simulink model "WPT_system_experimental_setup"  (R2022b)
settings: Solver=VariableStepAuto  StartTime=0.0  StopTime=0.030  RelTol=1e-3  EnableMultiTasking=on
InitFcn:
  | % Global param
  | f0 = 85000;
  | V_dc = 10;
  | Max_c = 5;
  | rise_time = 3e-3;
  | 
  | % Zed board ADC param
  | ADC_max_amp = 40;
  | ADC_max_vol = 1.25;
  | ADC_f_sample = 1e6;
  | ADC_bits = 12;
  | 
  | % Primary param
  | L1 = 24e-6;
  | C1 = 138e-9; %1/((2*pi*f0)^2*L1);
  | R1 = 0.075;
  | 
  | 
  | % Secondary param
  | M = 1.6e-6;
  | L2 = 24e-6;
  | C2 = 141e-9;% 1/((2*pi*f0)^2*L2);
  | 
  | R2 = 0.075;
  | R_l = 1.25;
  | C_out = 10e-6;
  | L_out = 1e-6;
  | 
  | % PRBS param
  | PRBS_n_bit = 10;
  | PRBS_f = f0*2; %1e5;
  | PRBS_up = 1; % pwm up time in %
  | PRBS_delay = 1.1* 1/(PRBS_f) * PRBS_up/100;
  | PRBS_amplitude = 0.1;
  | PRBS_n_period = 2;
  | PRBS_t_start = 0.0002 + PRBS_n_period * (2^(PRBS_n_bit) - 1)/PRBS_f;
  | PRBS_t_stop = 0.0002 + 2*PRBS_n_period * (2^(PRBS_n_bit) - 1)/PRBS_f;
  | transport_delay = PRBS_t_stop - PRBS_t_start;
  | 
  | 
  | % Emphasis filters param
  | 
  | f_z = 42000;
  | T_s_1 = 1/PRBS_f;
  | T_s_2 = 1/ADC_f_sample;
  | Filter_param_1 = exp(-2*pi*T_s_1 * f_z);
  | Filter_param_2 = exp(-2*pi*T_s_2 * f_z);
  | 
  | %Filter_param = 0.652296150979446; % 68000
model workspace (MAT data in the model file):
  C1 = Simulink.Parameter
  C1.Value = 4.1e-08
  C1.DataType = 'auto'
  C1.Complexity = 'real'
  C1.Dimensions = [1 1]
  C2 = Simulink.Parameter
  C2.Value = 4.2e-08
  C2.DataType = 'auto'
  C2.Complexity = 'real'
  C2.Dimensions = [1 1]
  C_out = Simulink.Parameter
  C_out.Value = 1e-05
  C_out.DataType = 'auto'
  C_out.Complexity = 'real'
  C_out.Dimensions = [1 1]
  L1 = Simulink.Parameter
  L1.Value = 8.6e-05
  L1.DataType = 'auto'
  L1.Complexity = 'real'
  L1.Dimensions = [1 1]
  L2 = Simulink.Parameter
  L2.Value = 8.4e-05
  L2.DataType = 'auto'
  L2.Complexity = 'real'
  L2.Dimensions = [1 1]
  M = Simulink.Parameter
  M.Value = 7e-06
  M.DataType = 'auto'
  M.Complexity = 'real'
  M.Dimensions = [1 1]
  R1 = Simulink.Parameter
  R1.Value = 0.35
  R1.DataType = 'auto'
  R1.Complexity = 'real'
  R1.Dimensions = [1 1]
  R2 = Simulink.Parameter
  R2.Value = 0.3
  R2.DataType = 'auto'
  R2.Complexity = 'real'
  R2.Dimensions = [1 1]
  R_l = Simulink.Parameter
  R_l.Value = 2
  R_l.DataType = 'auto'
  R_l.Complexity = 'real'
  R_l.Dimensions = [1 1]
  V_dc = Simulink.Parameter
  V_dc.Value = 400
  V_dc.DataType = 'auto'
  V_dc.Complexity = 'real'
  V_dc.Dimensions = [1 1]
  f0 = Simulink.Parameter
  f0.Value = 85000
  f0.DataType = 'auto'
  f0.Complexity = 'real'
  f0.Dimensions = [1 1]
  mwTaskManagerKernelLatency = 0
undefined symbols (not defined in the file or in its folder): plecs
libraries: simulink_extras x36, simulink x6, hdlsllib x3, msbAdcArchitectures x2, plecslib_extras2 x2, slpidlib x2
CloseFcn:
  | % Define the command to call the Python script
  | pythonScript = 'cross_correlation.py';
  | command = ['python ', pythonScript];
  | 
  | % Execute the Python script
  | system(command);
settings Model: Creator=thoma  LastModifiedBy=thoma
settings SolverCC: PositivePriorityOrder=on
settings OptimizationCC: EnhancedBackFolding=on  PassReuseOutputArgsAs=Individual arguments  ZeroExternalMemoryAtStartup=off  ZeroInternalMemoryAtStartup=off  MaxStackSize=64  OptimizeBlockOrder=speed  DifferentSizesBufferReuse=on  OptimizationCustomize=off  EfficientTunableParamExpr=on
settings DebuggingCC: ParameterTunabilityLossMsg=error
settings HardwareCC: ProdBitPerPointer=32  ProdBitPerSizeT=32  ProdBitPerPtrDiffT=32  ProdLargestAtomicInteger=Long  ProdLargestAtomicFloat=Double  ProdWordSize=32  ProdHWDeviceType=ARM Compatible->ARM Cortex  HardwareBoardFeatureSet=SoCBlockset
settings ModelReferenceCC: ModelReferenceNumInstancesAllowed=Single
settings SFSimCC: MATLABDynamicMemAlloc=off
settings RTWCC: Description=Embedded Coder  SystemTargetFile=ert.tlc  HardwareBoard=ZedBoard  TLCOptions="-aInlineSetEventsForThisBaseRateFcn=TLC_FALSE -aSuppressMultiTaskScheduler=TLC_FALSE  -aRateBasedStepFcn=0"  TemplateMakefile=ert_default_tmf
settings CodeAppCC: ForceParamTrailComments=on  IgnoreCustomStorageClasses=off  OperatorAnnotations=on  SimulinkDataObjDesc=on  SFDataObjDesc=on  InsertBlockDesc=on

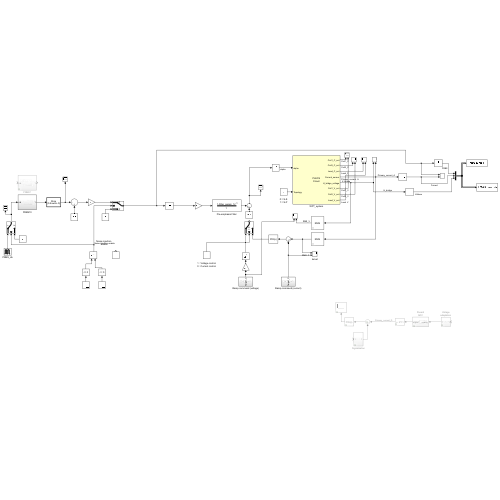
[thumbnail: Simulink's stored preview of the top-level diagram]
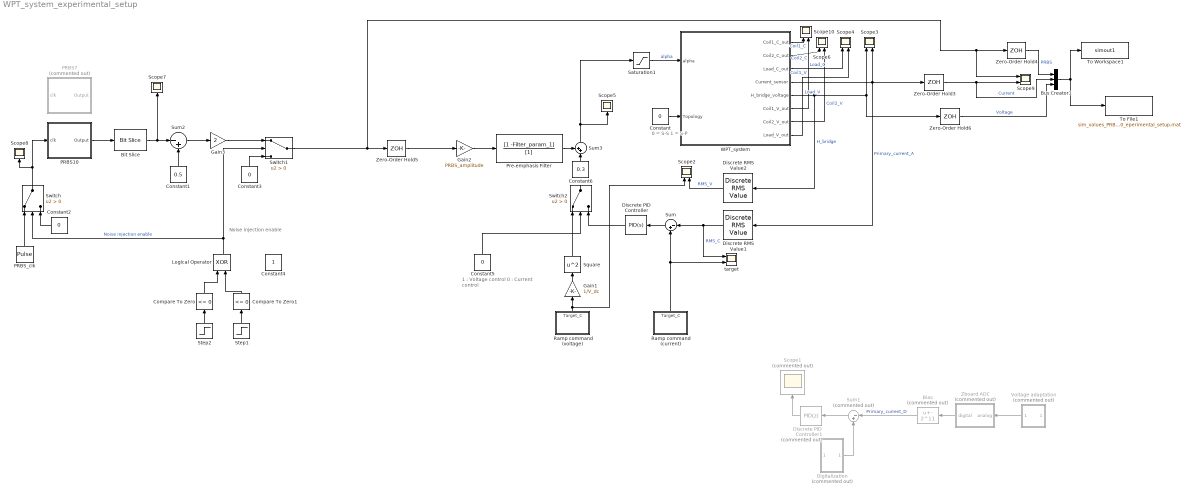
== system WPT_system_experimental_setup ==
  note: 0 = S-S
      | 1 = S-P
  note: Noise injection
      | enable
  note: 1 : Voltage control
      | 0 : Current control
  Bias : Bias  Commented=on  Bias=- 2^11  SaturateOnIntegerOverflow=off
  Bit Slice : hdlsllib/Logic and Bit Operations/Bit Slice  lidx=0  ridx=0
  Bus Creator1 : BusCreator  Inputs=3
  Compare To Zero : simulink/Logic and Bit Operations/Compare To Zero  relop=<=  OutDataTypeStr=boolean
  Compare To Zero1 : simulink/Logic and Bit Operations/Compare To Zero  relop=<=  OutDataTypeStr=boolean
  Constant{,2..3,5} (4 alike) : Constant  Value=0
  Constant1 : Constant  Value=0.5
  Constant4 : Constant
  Constant6 : Constant  Value=0.3
  Digitalization : Subsystem  Commented=on
  Discrete RMS Value1 : plecslib_extras2/Discrete Analysis/Discrete RMS Value  init=0  Ts=1/(30 * f0)  samples=60
      settings: SourceProductName=PLECS Extras
  Discrete RMS Value2 : plecslib_extras2/Discrete Analysis/Discrete RMS Value  init=0  Ts=1/(400 * f0)  samples=400
      settings: SourceProductName=PLECS Extras
  Discrete PID Controller : slpidlib/PID Controller  Controller=PID  Form=Parallel  TimeDomain=Continuous-time  UseExternalTs=off  SampleTime=-1  IntegratorMethod=Forward Euler  FilterMethod=Forward Euler  ControllerParametersSource=internal  P=0.075  I=5000  UseKiTs=off  D=0  N=100  UseFilter=on  TunerSelectOption=Transfer Function Based (PID Tuner App)  InitialConditionSource=internal  InitialConditionForIntegrator=0  InitialConditionForFilter=0  DifferentiatorICPrevScaledInput=0  ExternalReset=none  TrackingMode=off  Kt=1  LimitOutput=off  SatLimitsSource=internal  UpperSaturationLimit=inf  LowerSaturationLimit=-inf  LinearizeAsGain=off  AntiWindupMode=none  Kb=1  LimitIntegrator=off  UpperIntegratorSaturationLimit=inf  LowerIntegratorSaturationLimit=-inf  POutMin=[]  POutMax=[]  IOutMin=[]  IOutMax=[]  DOutMin=[]  DOutMax=[]  NOutMin=[]  NOutMax=[]  SumOutMin=[]  SumOutMax=[]  SaturationOutMin=[]  SaturationOutMax=[]  PParamMin=[]  PParamMax=[]  IParamMin=[]  IParamMax=[]  DParamMin=[]  DParamMax=[]  NParamMin=[]  NParamMax=[]  KbParamMin=[]  KbParamMax=[]  KtParamMin=[]  KtParamMax=[]  KbOutMin=[]  KbOutMax=[]  KtOutMin=[]  KtOutMax=[]  IntegratorOutMin=[]  IntegratorOutMax=[]  FilterOutMin=[]  FilterOutMax=[]  SumI1OutMin=[]  SumI1OutMax=[]  SumI2OutMin=[]  SumI2OutMax=[]  SumI3OutMin=[]  SumI3OutMax=[]  SumI4OutMin=[]  SumI4OutMax=[]  SumDOutMin=[]  SumDOutMax=[]  DifferentiatorOutMin=[]  DifferentiatorOutMax=[]  FilterDiffOutCoefMin=[]  FilterDiffOutCoefMax=[]  ReciprocalOutMin=[]  ReciprocalOutMax=[]  SumDenOutMin=[]  SumDenOutMax=[]  SumNumOutMin=[]  SumNumOutMax=[]  DivideOutMin=[]  DivideOutMax=[]  UdiffTsProdOutMin=[]  UdiffTsProdOutMax=[]  NTsProdOutMin=[]  NTsProdOutMax=[]  UintegralTsProdOutMin=[]  UintegralTsProdOutMax=[]  UngainTsProdOutMin=[]  UngainTsProdOutMax=[]  ClampingZeroOutDataTypeStr=Inherit: Inherit via back propagation  ClampingZeroOutMin=[]  ClampingZeroOutMax=[]  FilterDenConstantOutDataTypeStr=Inherit: Inherit via back propagation  FilterDenConstantOutMin=[]  FilterDenConstantOutMax=[]  PCopyOutDataTypeStr=Inherit: Inherit via back propagation  PCopyOutMin=[]  PCopyOutMax=[]  NCopyOutDataTypeStr=Inherit: Inherit via back propagation  NCopyOutMin=[]  NCopyOutMax=[]  IntegratorContinuousStateAttributes=''  IntegratorStateMustResolveToSignalObject=off  IntegratorRTWStateStorageClass=Auto  FilterContinuousStateAttributes=''  FilterStateMustResolveToSignalObject=off  FilterRTWStateStorageClass=Auto  ParallelPVariant=InternalParameters  IdealPVariant=Disabled  IVariant=InternalParameters  DVariant=InternalParameters  IntegratorVariant=Continuous  SatVariant=Disabled  AWVariant=Passthrough  PCopyVariant=Disabled  TRVariant=Disabled  FdbkBlocksVariant=Forward  IdealPFdbkVariant=Disabled  SatFdbkVariant=Disabled  DerivativeFilterVariant=ContFilter  NVariant=InternalParameters  NCopyVariant=Disabled  FilterICVariant=InternalICsFilter  IntegratorICVariant=InternalICs  ExternalResetVariant=Disabled  TRSumVariant=Passthrough  SumFdbkVariant=Disabled  SumVariant=Sum_PID  TsampFilterVariant=InternalTs  TsampNgainVariant=Passthrough  TsampIntegralVariant=Passthrough  ExternalSaturationOutDataTypeStr=Inherit: Same as second input
      settings: LibrarySourceBlock=hdlsllib/Discrete/Discrete PID Controller
  Discrete PID Controller1 : slpidlib/PID Controller  Commented=on  Controller=PID  Form=Parallel  TimeDomain=Discrete-time  UseExternalTs=off  SampleTime=-1  IntegratorMethod=Forward Euler  FilterMethod=Forward Euler  ControllerParametersSource=internal  P=24  I=0  UseKiTs=off  D=0  N=100  UseFilter=on  TunerSelectOption=Transfer Function Based (PID Tuner App)  InitialConditionSource=internal  InitialConditionForIntegrator=0  InitialConditionForFilter=0  DifferentiatorICPrevScaledInput=0  ExternalReset=none  TrackingMode=off  Kt=1  LimitOutput=off  SatLimitsSource=internal  UpperSaturationLimit=inf  LowerSaturationLimit=-inf  LinearizeAsGain=off  AntiWindupMode=none  Kb=1  LimitIntegrator=off  UpperIntegratorSaturationLimit=inf  LowerIntegratorSaturationLimit=-inf  POutMin=[]  POutMax=[]  IOutMin=[]  IOutMax=[]  DOutMin=[]  DOutMax=[]  NOutMin=[]  NOutMax=[]  SumOutMin=[]  SumOutMax=[]  SaturationOutMin=[]  SaturationOutMax=[]  PParamMin=[]  PParamMax=[]  IParamMin=[]  IParamMax=[]  DParamMin=[]  DParamMax=[]  NParamMin=[]  NParamMax=[]  KbParamMin=[]  KbParamMax=[]  KtParamMin=[]  KtParamMax=[]  KbOutMin=[]  KbOutMax=[]  KtOutMin=[]  KtOutMax=[]  IntegratorOutMin=[]  IntegratorOutMax=[]  FilterOutMin=[]  FilterOutMax=[]  SumI1OutMin=[]  SumI1OutMax=[]  SumI2OutMin=[]  SumI2OutMax=[]  SumI3OutMin=[]  SumI3OutMax=[]  SumI4OutMin=[]  SumI4OutMax=[]  SumDOutMin=[]  SumDOutMax=[]  DifferentiatorOutMin=[]  DifferentiatorOutMax=[]  FilterDiffOutCoefMin=[]  FilterDiffOutCoefMax=[]  ReciprocalOutMin=[]  ReciprocalOutMax=[]  SumDenOutMin=[]  SumDenOutMax=[]  SumNumOutMin=[]  SumNumOutMax=[]  DivideOutMin=[]  DivideOutMax=[]  UdiffTsProdOutMin=[]  UdiffTsProdOutMax=[]  NTsProdOutMin=[]  NTsProdOutMax=[]  UintegralTsProdOutMin=[]  UintegralTsProdOutMax=[]  UngainTsProdOutMin=[]  UngainTsProdOutMax=[]  ClampingZeroOutDataTypeStr=Inherit: Inherit via back propagation  ClampingZeroOutMin=[]  ClampingZeroOutMax=[]  FilterDenConstantOutDataTypeStr=Inherit: Inherit via back propagation  FilterDenConstantOutMin=[]  FilterDenConstantOutMax=[]  PCopyOutDataTypeStr=Inherit: Inherit via back propagation  PCopyOutMin=[]  PCopyOutMax=[]  NCopyOutDataTypeStr=Inherit: Inherit via back propagation  NCopyOutMin=[]  NCopyOutMax=[]  IntegratorContinuousStateAttributes=''  IntegratorStateMustResolveToSignalObject=off  IntegratorRTWStateStorageClass=Auto  FilterContinuousStateAttributes=''  FilterStateMustResolveToSignalObject=off  FilterRTWStateStorageClass=Auto  ParallelPVariant=InternalParameters  IdealPVariant=Disabled  IVariant=InternalParameters  DVariant=InternalParameters  IntegratorVariant=Discrete  SatVariant=Disabled  AWVariant=Passthrough  PCopyVariant=Disabled  TRVariant=Disabled  FdbkBlocksVariant=Forward  IdealPFdbkVariant=Disabled  SatFdbkVariant=Disabled  DerivativeFilterVariant=ForwardEulerFilter  NVariant=InternalParameters  NCopyVariant=Disabled  FilterICVariant=InternalICsFilter  IntegratorICVariant=InternalICs  ExternalResetVariant=Disabled  TRSumVariant=Passthrough  SumFdbkVariant=Disabled  SumVariant=Sum_PID  TsampFilterVariant=InternalTs  TsampNgainVariant=Passthrough  TsampIntegralVariant=Passthrough  ExternalSaturationOutDataTypeStr=Inherit: Same as second input
      settings: LibrarySourceBlock=hdlsllib/Discrete/Discrete PID Controller
  Gain1 : Gain  Gain=1/V_dc
  Gain2 : Gain  Gain=PRBS_amplitude
  Gain3 : Gain  Gain=2
  Logical Operator : Logic  Operator=XOR  AllPortsSameDT=off  OutDataTypeStr=boolean
  PRBS10 : Subsystem
  PRBS7 : Subsystem  Commented=on
  "PRBS_clk " : DiscretePulseGenerator  PulseType=Time based  Period=1/PRBS_f  PulseWidth=PRBS_up
  Pre-emphasis Filter : DiscreteFilter  Numerator=[1 -Filter_param_1]  Denominator=[1]
  Ramp command (current) : Subsystem
  Ramp command (voltage) : Subsystem
  Saturation1 : Saturate  UpperLimit=1  LowerLimit=0
  Scope1 : Scope  Commented=on
  Scope{2..4,6,9..10} (6 alike) : Scope  NumInputPorts=2
  Scope5 : Scope
  Scope7 : Scope
  Scope8 : Scope
  Square : Math  Operator=square  SignedPower=on  RndMeth=Zero
  Step1 : Step  Time=PRBS_t_start  Before=1  After=0  SampleTime=0
  Step2 : Step  Time=PRBS_t_stop  Before=1  After=0  SampleTime=0
  Sum : Sum  Inputs=|-+
  Sum1 : Sum  Commented=on  Inputs=|-+
  Sum2 : Sum  Inputs=|-+  AccumDataTypeStr=double
  Sum3 : Sum  Inputs=++|
  Switch : Switch  Criteria=u2 > Threshold  SaturateOnIntegerOverflow=off  InputSameDT=off
  Switch1 : Switch  Criteria=u2 > Threshold  SaturateOnIntegerOverflow=off  InputSameDT=off
  Switch2 : Switch  Criteria=u2 > Threshold  SaturateOnIntegerOverflow=off  InputSameDT=off
  To File1 : ToFile  Filename=sim_values_PRBS10_eperimental_setup.mat  MatrixName=values  SampleTime=1e-6
  To Workspace1 : ToWorkspace  VariableName=simout1  SampleTime=1e-6
  Voltage adaptation : Subsystem  Commented=on
  WPT_system : Subsystem  LoadFcn=plecs('sl', 200);  InitFcn=plecs('sl', 214);  StartFcn=plecs('sl', 208);  StopFcn=plecs('sl', 209);  mask(PlecsCircuit){PLECSData=<binary blob, 4092 chars, not shown>}
      mask prompts: PLECSData "PLECS Data (Do not delete or modify!)"
      mask init:
      | % PLACE CUSTOM INITIALIZATIONS ABOVE
      | % DO NOT REMOVE
      | plecs('sl', 215);
      | % DO NOT REMOVE
      settings: CopyFcn=plecs('sl', 203);  DeleteFcn=plecs('sl', 205);  UndoDeleteFcn=plecs('sl', 206);  PreSaveFcn=plecs('sl', 211);  PostSaveFcn=plecs('sl', 201);  NameChangeFcn=plecs('sl', 210);  DestroyFcn=plecs('sl', 207);  PreCopyFcn=plecs('sl', 216);  OpenFcn=plecs('sl', 202);  ErrorFcn=plerrorfcn
      mask Help: eval('plecs(''help'', ''qthelp:///creatingacircuit.html'')')
      mask Display: disp('PLECS\nCircuit')
  Zboard ADC : Subsystem  Commented=on
  Zero-Order Hold3 : ZeroOrderHold  SampleTime=1/ADC_f_sample
  Zero-Order Hold4 : ZeroOrderHold  SampleTime=1e-6
  Zero-Order Hold5 : ZeroOrderHold  SampleTime=1/PRBS_f
  Zero-Order Hold6 : ZeroOrderHold  SampleTime=1/ADC_f_sample
  target : Scope  NumInputPorts=2
  wires:
  Constant/1 -> WPT_system/2(Topology)
  Sum/1 -> Discrete PID Controller/1
  Discrete RMS Value1/1 -> Sum/1, target/1  "RMS_C"
  Bit Slice/1 -> Scope7/1, Sum2/1
  Ramp command (current)/1(Target_C) -> Sum/2, target/2
  Bias/1 -> Sum1/1  "Primary_current_D"
  Voltage adaptation/1(Out1) -> Zboard ADC/1(analog)
  Zboard ADC/1(digital) -> Bias/1
  Digitalization/1(Output) -> Sum1/2
  Sum1/1 -> Discrete PID Controller1/1
  Discrete PID Controller1/1 -> Scope1/1
  Ramp command (voltage)/1(Target_C) -> Scope2/1, Gain1/1
  Gain1/1 -> Square/1
  Constant1/1 -> Sum2/2
  Sum2/1 -> Gain3/1
  Saturation1/1 -> WPT_system/1(alpha)  "alpha"
  WPT_system/3(Load_C_out) -> Scope4/1  "Load_C"
  WPT_system/8(Load_V_out) -> Scope4/2  "Load_V"
  WPT_system/2(Coil2_C_out) -> Scope6/1  "Coil2_C"
  WPT_system/7(Coil2_V_out) -> Scope6/2  "Coil2_V"
  Square/1 -> Switch2/1
  Discrete PID Controller/1 -> Switch2/3
  Constant5/1 -> Switch2/2
  Logical Operator/1 -> Switch/2, Switch1/2  "Noise injection enable"
  "PRBS_clk "/1 -> Switch/1
  Constant2/1 -> Switch/3
  Constant3/1 -> Switch1/3
  Gain3/1 -> Switch1/1
  Discrete RMS Value2/1 -> Scope2/2  "RMS_V"
  Sum3/1 -> Scope5/1, Saturation1/1
  PRBS10/1(Output) -> Bit Slice/1
  Switch/1 -> PRBS10/1(clk), Scope8/1
  Constant6/1 -> Sum3/2
  Step2/1 -> Compare To Zero/1
  Step1/1 -> Compare To Zero1/1
  Compare To Zero/1 -> Logical Operator/1
  Compare To Zero1/1 -> Logical Operator/2
  Pre-emphasis Filter/1 -> Sum3/1
  Gain2/1 -> Pre-emphasis Filter/1
  Zero-Order Hold5/1 -> Gain2/1
  Bus Creator1/1 -> To File1/1, To Workspace1/1
  Zero-Order Hold6/1 -> Bus Creator1/3  "Voltage"
  WPT_system/5(H_bridge_voltage) -> Zero-Order Hold6/1, Scope3/1, Discrete RMS Value2/1  "H_bridge"
  Zero-Order Hold4/1 -> Bus Creator1/1  "PRBS"
  Switch1/1 -> Scope9/1, Zero-Order Hold4/1, Zero-Order Hold5/1
  Zero-Order Hold3/1 -> Bus Creator1/2, Scope9/2  "Current"
  WPT_system/4(Current_sensor) -> Zero-Order Hold3/1, Discrete RMS Value1/1, Scope3/2  "Primary_current_A"
  WPT_system/1(Coil1_C_out) -> Scope10/1  "Coil1_C"
  WPT_system/6(Coil1_V_out) -> Scope10/2  "Coil1_V"

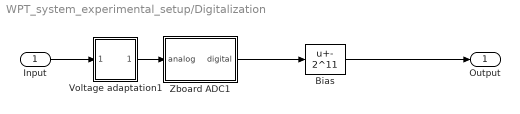
== system WPT_system_experimental_setup/Digitalization ==
  Input : Inport
  Bias : Bias  Bias=- 2^11  SaturateOnIntegerOverflow=off
  Voltage adaptation1 : Subsystem
  Zboard ADC1 : Subsystem
  Output : Outport
  wires:
  Voltage adaptation1/1(Out1) -> Zboard ADC1/1(analog)
  Input/1 -> Voltage adaptation1/1(In1)
  Zboard ADC1/1(digital) -> Bias/1
  Bias/1 -> Output/1

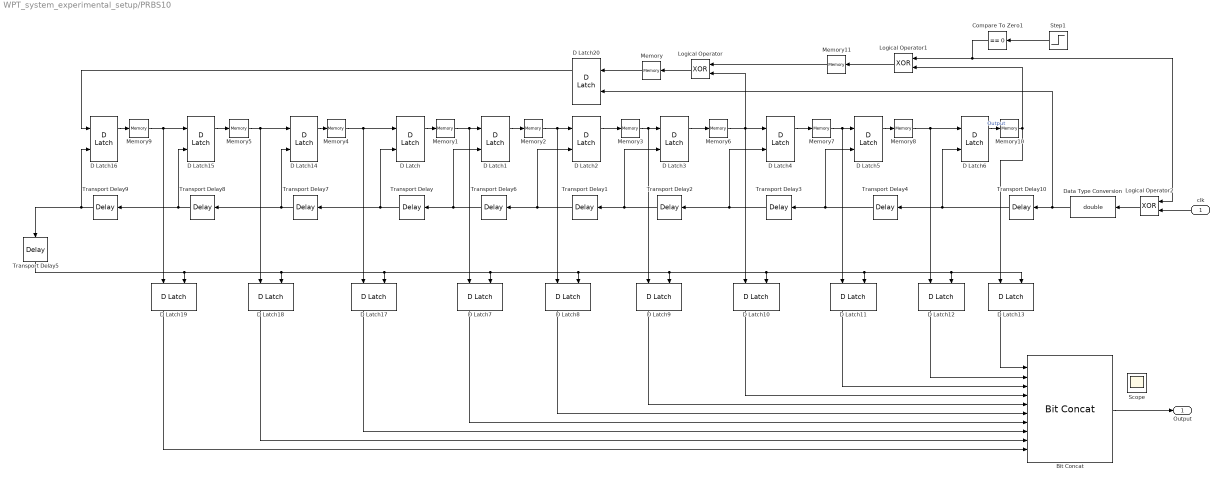
== system WPT_system_experimental_setup/PRBS10 ==
  clk : Inport
  Bit Concat : hdlsllib/Logic and Bit Operations/Bit Concat  numInputs=10
  Compare To Zero1 : simulink/Logic and Bit Operations/Compare To Zero  relop===  OutDataTypeStr=boolean
  D Latch{,1..20} (21 alike) : simulink_extras/Flip Flops/D Latch
  Data Type Conversion : DataTypeConversion  OutDataTypeStr=double  SaturateOnIntegerOverflow=off  RndMeth=Floor
  Logical Operator : Logic  Operator=XOR  AllPortsSameDT=off  OutDataTypeStr=boolean
  Logical Operator1 : Logic  Operator=XOR  AllPortsSameDT=off  OutDataTypeStr=boolean
  Logical Operator2 : Logic  Operator=XOR  AllPortsSameDT=off
  Memory{,1..11} (12 alike) : Memory
  Scope : Scope
  Step1 : Step  Time=1* PRBS_delay  SampleTime=0
  Transport Delay{,1..4,6..10} (10 alike) : TransportDelay  DelayTime=PRBS_delay  BufferSize=16384
  Transport Delay5 : TransportDelay  DelayTime=PRBS_delay  InitialOutput=1  BufferSize=16384
  Output : Outport
  wires:
  Transport Delay1/1 -> D Latch2/2, Transport Delay6/1
  Transport Delay4/1 -> D Latch5/2, Transport Delay3/1
  Transport Delay2/1 -> D Latch3/2, Transport Delay1/1
  Transport Delay3/1 -> D Latch4/2, Transport Delay2/1
  D Latch1/1 -> Memory2/1
  D Latch/1 -> Memory1/1
  D Latch2/1 -> Memory3/1
  Logical Operator/1 -> Memory/1
  D Latch4/1 -> Memory7/1
  D Latch3/1 -> Memory6/1
  Bit Concat/1 -> Output/1
  D Latch5/1 -> Memory8/1
  Transport Delay6/1 -> D Latch1/2, Transport Delay/1
  Memory3/1 -> D Latch3/1, D Latch9/1
  D Latch6/1 -> Memory10/1  "Output"
  D Latch13/1 -> Bit Concat/1
  D Latch12/1 -> Bit Concat/2
  D Latch11/1 -> Bit Concat/3
  D Latch10/1 -> Bit Concat/4
  D Latch9/1 -> Bit Concat/5
  D Latch8/1 -> Bit Concat/6
  D Latch7/1 -> Bit Concat/7
  Transport Delay/1 -> Transport Delay7/1, D Latch/2
  D Latch15/1 -> Memory5/1
  Transport Delay7/1 -> Transport Delay8/1, D Latch14/2
  D Latch16/1 -> Memory9/1
  Transport Delay9/1 -> Transport Delay5/1, D Latch16/2
  Transport Delay8/1 -> Transport Delay9/1, D Latch15/2
  Transport Delay5/1 -> D Latch19/2, D Latch18/2, D Latch17/2, D Latch9/2, D Latch10/2, D Latch11/2, D Latch13/2, D Latch12/2, D Latch8/2, D Latch7/2
  D Latch17/1 -> Bit Concat/8
  D Latch18/1 -> Bit Concat/9
  D Latch19/1 -> Bit Concat/10
  Memory2/1 -> D Latch2/1, D Latch8/1
  Memory7/1 -> D Latch11/1, D Latch5/1
  Memory8/1 -> D Latch6/1, D Latch12/1
  Memory1/1 -> D Latch1/1, D Latch7/1
  Memory9/1 -> D Latch19/1, D Latch15/1
  D Latch14/1 -> Memory4/1
  Memory4/1 -> D Latch/1, D Latch17/1
  Memory6/1 -> Logical Operator/2, D Latch4/1, D Latch10/1
  Memory5/1 -> D Latch18/1, D Latch14/1
  Step1/1 -> Compare To Zero1/1
  Compare To Zero1/1 -> Logical Operator2/1, Logical Operator1/1
  Logical Operator1/1 -> Memory11/1
  Memory10/1 -> D Latch13/1, Logical Operator1/2
  Memory11/1 -> Logical Operator/1
  Memory/1 -> D Latch20/1
  D Latch20/1 -> D Latch16/1
  Transport Delay10/1 -> D Latch6/2, Transport Delay4/1
  Logical Operator2/1 -> Data Type Conversion/1
  clk/1 -> Logical Operator2/2
  Data Type Conversion/1 -> D Latch20/2, Transport Delay10/1

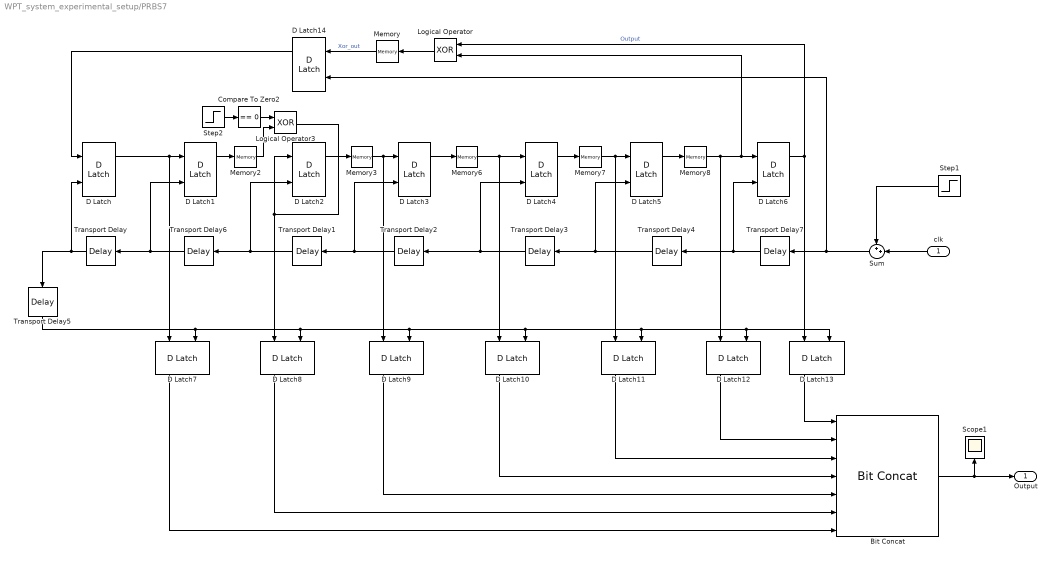
== system WPT_system_experimental_setup/PRBS7 ==
  clk : Inport
  Bit Concat : hdlsllib/Logic and Bit Operations/Bit Concat  numInputs=7
  Compare To Zero2 : simulink/Logic and Bit Operations/Compare To Zero  relop===  OutDataTypeStr=boolean
  D Latch{,1..14} (15 alike) : simulink_extras/Flip Flops/D Latch
  Logical Operator : Logic  Operator=XOR  AllPortsSameDT=off  OutDataTypeStr=boolean
  Logical Operator3 : Logic  Operator=XOR  AllPortsSameDT=off  OutDataTypeStr=boolean
  Memory{,2..3,6..8} (6 alike) : Memory
  Scope1 : Scope
  Step1 : Step  Time=5/(100*PRBS_f)  Before=1  After=0  SampleTime=0
  Step2 : Step  Time=6* PRBS_delay  SampleTime=0
  Sum : Sum  Inputs=++|
  Transport Delay{,1..4,6..7} (7 alike) : TransportDelay  DelayTime=PRBS_delay  BufferSize=16384
  Transport Delay5 : TransportDelay  DelayTime=PRBS_delay  InitialOutput=1  BufferSize=16384
  Output : Outport
  wires:
  D Latch10/1 -> Bit Concat/4
  D Latch7/1 -> Bit Concat/7
  Transport Delay5/1 -> D Latch9/2, D Latch10/2, D Latch11/2, D Latch13/2, D Latch12/2, D Latch8/2, D Latch7/2
  Transport Delay1/1 -> D Latch2/2, Transport Delay6/1
  Transport Delay4/1 -> D Latch5/2, Transport Delay3/1
  Transport Delay2/1 -> D Latch3/2, Transport Delay1/1
  Transport Delay/1 -> Transport Delay5/1, D Latch/2
  D Latch8/1 -> Bit Concat/6
  Transport Delay3/1 -> D Latch4/2, Transport Delay2/1
  D Latch1/1 -> Memory2/1
  D Latch/1 -> D Latch1/1, D Latch7/1
  D Latch2/1 -> Memory3/1
  Memory7/1 -> D Latch5/1, D Latch11/1
  Logical Operator/1 -> Memory/1
  D Latch4/1 -> Memory7/1
  D Latch3/1 -> Memory6/1
  Bit Concat/1 -> Output/1, Scope1/1
  Memory2/1 -> Logical Operator3/2
  D Latch5/1 -> Memory8/1
  Compare To Zero2/1 -> Logical Operator3/1
  Step2/1 -> Compare To Zero2/1
  Transport Delay6/1 -> D Latch1/2, Transport Delay/1
  Memory8/1 -> Logical Operator/2, D Latch6/1, D Latch12/1
  Memory6/1 -> D Latch4/1, D Latch10/1
  D Latch9/1 -> Bit Concat/5
  D Latch12/1 -> Bit Concat/2
  D Latch13/1 -> Bit Concat/1
  Memory3/1 -> D Latch3/1, D Latch9/1
  D Latch11/1 -> Bit Concat/3
  D Latch6/1 -> Logical Operator/1, D Latch13/1  "Output"
  Logical Operator3/1 -> D Latch2/1, D Latch8/1
  Memory/1 -> D Latch14/1  "Xor_out"
  D Latch14/1 -> D Latch/1
  Sum/1 -> D Latch14/2, Transport Delay7/1
  Transport Delay7/1 -> D Latch6/2, Transport Delay4/1
  Step1/1 -> Sum/1
  clk/1 -> Sum/2

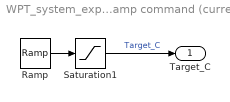
== system WPT_system_experimental_setup/Ramp command (current) ==
  Ramp : simulink/Sources/Ramp  slope=Max_c/rise_time  start=0  InitialOutput=0
  Saturation1 : Saturate  UpperLimit=Max_c  LowerLimit=0
  Target_C : Outport
  wires:
  Ramp/1 -> Saturation1/1
  Saturation1/1 -> Target_C/1  "Target_C"

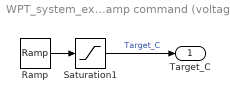
== system WPT_system_experimental_setup/Ramp command (voltage) ==
  Ramp : simulink/Sources/Ramp  slope=V_dc/(2*rise_time)  start=0  InitialOutput=0
  Saturation1 : Saturate  UpperLimit=V_dc/2  LowerLimit=0
  Target_C : Outport
  wires:
  Ramp/1 -> Saturation1/1
  Saturation1/1 -> Target_C/1  "Target_C"

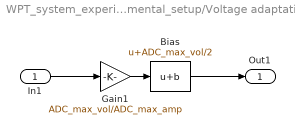
== system WPT_system_experimental_setup/Voltage adaptation ==
  In1 : Inport
  Bias : Bias  Bias=ADC_max_vol/2  SaturateOnIntegerOverflow=off
  Gain1 : Gain  Gain=ADC_max_vol/ADC_max_amp
  Out1 : Outport
  wires:
  Gain1/1 -> Bias/1
  In1/1 -> Gain1/1
  Bias/1 -> Out1/1

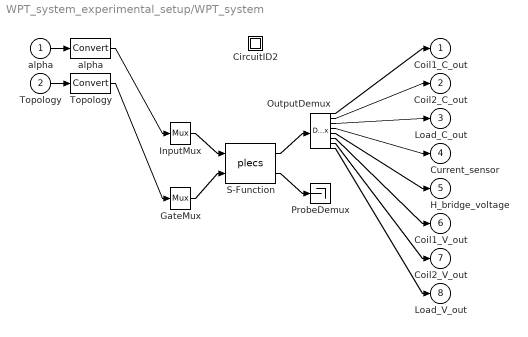
== system WPT_system_experimental_setup/WPT_system ==
  alpha : Inport  PortDimensions=1
  Topology : Inport  Port=2  PortDimensions=1
  " CircuitID2 " : Subsystem
  " GateMux " : Mux  Inputs=[ 1 ]
  " InputMux " : Mux  Inputs=[ 1 ]
  " OutputDemux " : Demux  Outputs=[ 1 1 1 1 1 1 1 1 ]
  " ProbeDemux " : Terminator
  " S-Function " : S-Function  FunctionName=plecs  SFunctionDeploymentMode=off  EnableBusSupport=off
  " Topology " : DataTypeConversion
  " alpha " : DataTypeConversion
  Coil1_C_out : Outport  PortDimensions=1
  Coil2_C_out : Outport  Port=2  PortDimensions=1
  Load_C_out : Outport  Port=3  PortDimensions=1
  Current_sensor : Outport  Port=4  PortDimensions=1
  H_bridge_voltage : Outport  Port=5  PortDimensions=1
  Coil1_V_out : Outport  Port=6  PortDimensions=1
  Coil2_V_out : Outport  Port=7  PortDimensions=1
  Load_V_out : Outport  Port=8  PortDimensions=1
  wires:
  " InputMux "/1 -> " S-Function "/1
  " GateMux "/1 -> " S-Function "/2
  " S-Function "/1 -> " OutputDemux "/1
  " S-Function "/2 -> " ProbeDemux "/1
  alpha/1 -> " alpha "/1
  " alpha "/1 -> " InputMux "/1
  Topology/1 -> " Topology "/1
  " Topology "/1 -> " GateMux "/1
  " OutputDemux "/1 -> Coil1_C_out/1
  " OutputDemux "/2 -> Coil2_C_out/1
  " OutputDemux "/3 -> Load_C_out/1
  " OutputDemux "/4 -> Current_sensor/1
  " OutputDemux "/5 -> H_bridge_voltage/1
  " OutputDemux "/6 -> Coil1_V_out/1
  " OutputDemux "/7 -> Coil2_V_out/1
  " OutputDemux "/8 -> Load_V_out/1

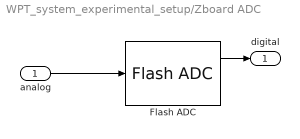
== system WPT_system_experimental_setup/Zboard ADC ==
  analog : Inport
  Flash ADC : msbAdcArchitectures/Flash ADC  LabelModeActiveChoice=Simulink Blocks  NBits=12  InputRange=[0 1.25]  ExtStartClk=off  StartFreq=ADC_f_sample  StartClkJitter=1e-12  SampleInterval=0.25e-6  Trigger=Rising edge  MatchScale=off  OutputPolarity=Auto  OutDataType=double  SimulateUsing=Simulink blocks  EnableImp=off  OffsetError=0  OffsetErrorUnit=LSB  GainError=0  GainErrorUnit=LSB  Bubbles=[]
  digital : Outport
  wires:
  Flash ADC/1 -> digital/1
  analog/1 -> Flash ADC/1

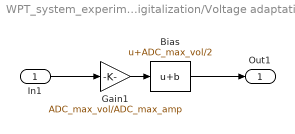
== system WPT_system_experimental_setup/Digitalization/Voltage adaptation1 ==
  In1 : Inport
  Bias : Bias  Bias=ADC_max_vol/2  SaturateOnIntegerOverflow=off
  Gain1 : Gain  Gain=ADC_max_vol/ADC_max_amp
  Out1 : Outport
  wires:
  Gain1/1 -> Bias/1
  In1/1 -> Gain1/1
  Bias/1 -> Out1/1

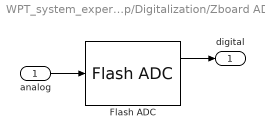
== system WPT_system_experimental_setup/Digitalization/Zboard ADC1 ==
  analog : Inport
  Flash ADC : msbAdcArchitectures/Flash ADC  LabelModeActiveChoice=Simulink Blocks  NBits=12  InputRange=[0 1.25]  ExtStartClk=off  StartFreq=ADC_f_sample  StartClkJitter=1e-12  SampleInterval=0.25e-6  Trigger=Rising edge  MatchScale=off  OutputPolarity=Auto  OutDataType=double  SimulateUsing=Simulink blocks  EnableImp=off  OffsetError=0  OffsetErrorUnit=LSB  GainError=0  GainErrorUnit=LSB  Bubbles=[]
  digital : Outport
  wires:
  Flash ADC/1 -> digital/1
  analog/1 -> Flash ADC/1

== system WPT_system_experimental_setup/WPT_system/ CircuitID2  ==
